simulink model "battery_thermal_model"  (R2024b)
settings: Solver=VariableStepAuto  StartTime=0.0  StopTime=10.0  RelTol=1e-3
model workspace (MAT data in the model file):
  C = 2
  R = 0.2
  Tenv = 25
  h = 5
settings Model: Creator=Nikhil M  LastModifiedBy=Nikhil M

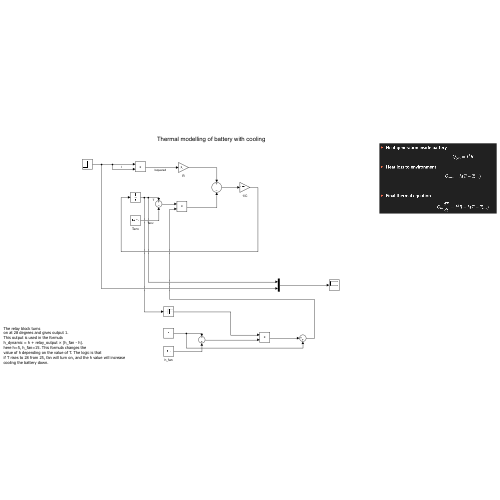
[thumbnail: Simulink's stored preview of the top-level diagram]
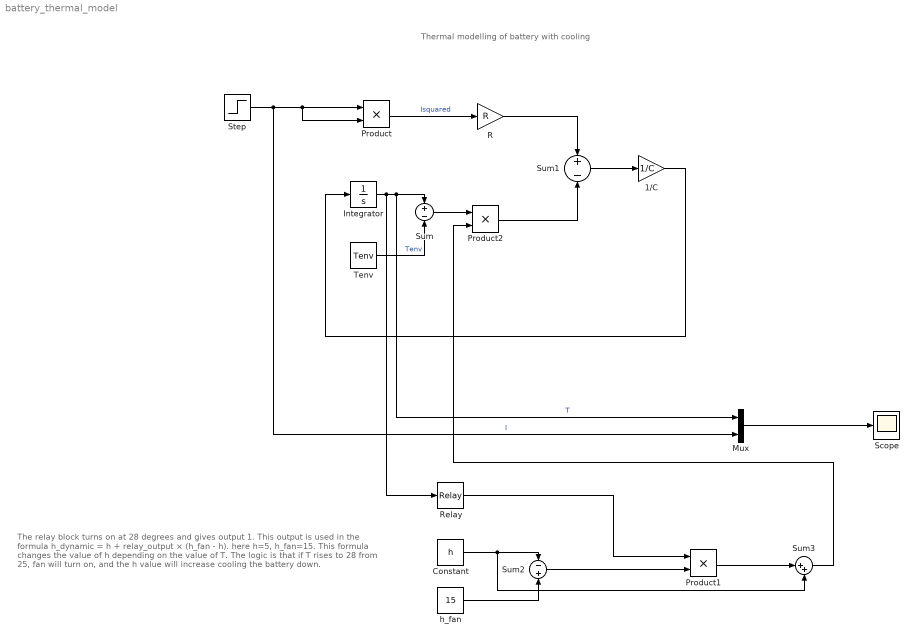
== system battery_thermal_model ==
  note: The relay block turns
      | on at 28 degrees and gives output 1.
      | This output is used in the formula
      | h_dynamic = h + relay_output × (h_fan - h).
      | here h=5, h_fan=15. This formula changes the
      | value of h depending on the value of T. The logic is that
      | if T rises to 28 from 25, fan will turn on, and the h value will increase
      | cooling the battery down.
  note: Thermal modelling of battery with cooling
  1/C : Gain  Gain=1/C
  Constant : Constant  Value=h
  Integrator : Integrator
  Mux : Mux  Inputs=2
  Product : Product
  Product1 : Product
  Product2 : Product
  R : Gain  Gain=R
  Relay : Relay  OnSwitchValue=28  OffSwitchValue=25
  Scope : Scope
  Step : Step  Time=5  Before=2  After=10  SampleTime=0
  Sum : Sum  Inputs=+|-
  Sum1 : Sum  Inputs=+|-
  Sum2 : Sum  Inputs=-|+
  Sum3 : Sum  Inputs=|++
  Tenv : Constant  Value=Tenv
  h_fan : Constant  Value=15
  wires:
  Step/1 -> Mux/2, Product/2, Product/1  "I"
  Product/1 -> R/1  "Isquared"
  Integrator/1 -> Relay/1, Mux/1, Sum/1  "T"
  Tenv/1 -> Sum/2  "Tenv"
  R/1 -> Sum1/1
  Sum1/1 -> 1/C/1
  1/C/1 -> Integrator/1
  Mux/1 -> Scope/1
  Sum/1 -> Product2/1
  Product2/1 -> Sum1/2
  Constant/1 -> Sum3/2, Sum2/1
  h_fan/1 -> Sum2/2
  Sum2/1 -> Product1/2
  Relay/1 -> Product1/1
  Product1/1 -> Sum3/1
  Sum3/1 -> Product2/2
